simulink subsystem "AC_OffsetRemover"  (R2024b)
settings: Solver=VariableStepAuto  StartTime=0.0  StopTime=10.0  RelTol=1e-3
settings Model: Creator=JesseJabezArendse  LastModifiedBy=JesseJabezArendse

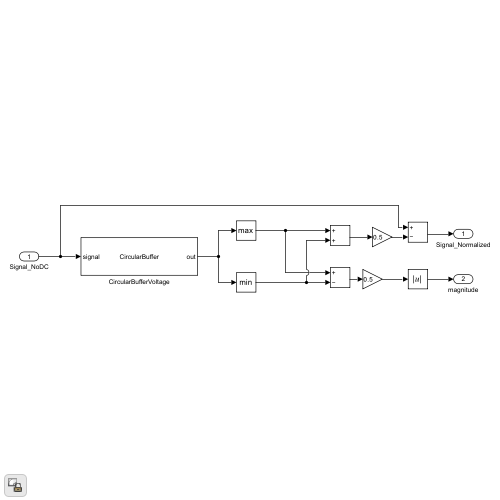
[thumbnail: Simulink's stored preview of the top-level diagram]
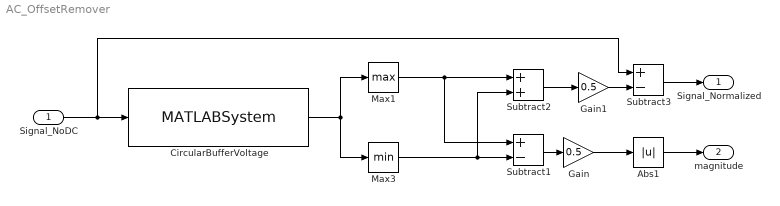
== system AC_OffsetRemover ==
  Signal_NoDC : Inport  OutDataTypeStr=single  PortDimensions=1
  Abs1 : Abs  SaturateOnIntegerOverflow=off
  CircularBufferVoltage : MATLABSystem  System=CircularBuffer  BufferLength=ADC_SamplingRate  InitialCondition=single( 0 )  SimulateUsing=Code generation
      mask Type: CircularBuffer
      mask Display:
      | disp('CircularBuffer');
      | port_label('input',1,'signal');
      | port_label('output',1,'out');
  Gain : Gain  Gain=0.5  OutDataTypeStr=single
  Gain1 : Gain  Gain=0.5  OutDataTypeStr=single
  Max1 : MinMax  Function=max  OutDataTypeStr=single
  Max3 : MinMax  OutDataTypeStr=single
  Subtract1 : Sum  Inputs=+-  OutDataTypeStr=single
  Subtract2 : Sum  OutDataTypeStr=single
  Subtract3 : Sum  Inputs=+-  OutDataTypeStr=single
  Signal_Normalized : Outport  OutDataTypeStr=single
  magnitude : Outport  Port=2  OutDataTypeStr=single
  wires:
  Signal_NoDC/1 -> Subtract3/1, CircularBufferVoltage/1
  Gain/1 -> Abs1/1
  Gain1/1 -> Subtract3/2
  CircularBufferVoltage/1 -> Max1/1, Max3/1
  Max3/1 -> Subtract1/2, Subtract2/2
  Max1/1 -> Subtract2/1, Subtract1/1
  Subtract1/1 -> Gain/1
  Subtract2/1 -> Gain1/1
  Subtract3/1 -> Signal_Normalized/1
  Abs1/1 -> magnitude/1
